simulink model "EngPrt_TrqLimPTO1"  (R2016b)
settings: configuration reference "CodeGenConfigSet" (kept outside this file)
values from neighbouring files (symbols this model uses):
  EngPrt_facPTOLim0_CUR = Calibration.Parameter    [init_EngPrt_TrqLimPTO.m]    (also in init_EngPrt_TrqLimPTO_SIL.m = Simulink.Parameter)
  EngPrt_facPTOLim0_CURX = Calibration.Parameter    [init_EngPrt_TrqLimPTO.m]    (also in init_EngPrt_TrqLimPTO_SIL.m = Simulink.Parameter)
  EngPrt_facPTOLim1_CUR = Calibration.Parameter    [init_EngPrt_TrqLimPTO.m]    (also in init_EngPrt_TrqLimPTO_SIL.m = Simulink.Parameter)
  EngPrt_facPTOLim1_CURX = Calibration.Parameter    [init_EngPrt_TrqLimPTO.m]    (also in init_EngPrt_TrqLimPTO_SIL.m = Simulink.Parameter)
  EngPrt_facPTOLim2_CUR = Calibration.Parameter    [init_EngPrt_TrqLimPTO.m]    (also in init_EngPrt_TrqLimPTO_SIL.m = Simulink.Parameter)
  EngPrt_facPTOLim2_CURX = Calibration.Parameter    [init_EngPrt_TrqLimPTO.m]    (also in init_EngPrt_TrqLimPTO_SIL.m = Simulink.Parameter)
  EngPrt_facPTOLim3_CUR = Calibration.Parameter    [init_EngPrt_TrqLimPTO.m]    (also in init_EngPrt_TrqLimPTO_SIL.m = Simulink.Parameter)
  EngPrt_facPTOLim3_CURX = Calibration.Parameter    [init_EngPrt_TrqLimPTO.m]    (also in init_EngPrt_TrqLimPTO_SIL.m = Simulink.Parameter)
  EngPrt_facPTOLim4_CUR = Calibration.Parameter    [init_EngPrt_TrqLimPTO.m]    (also in init_EngPrt_TrqLimPTO_SIL.m = Simulink.Parameter)
  EngPrt_facPTOLim4_CURX = Calibration.Parameter    [init_EngPrt_TrqLimPTO.m]    (also in init_EngPrt_TrqLimPTO_SIL.m = Simulink.Parameter)
settings Model: Creator=lenovo  LastModifiedBy=lenovo
settings ConfigSetRef: SourceLocation=Base Workspace

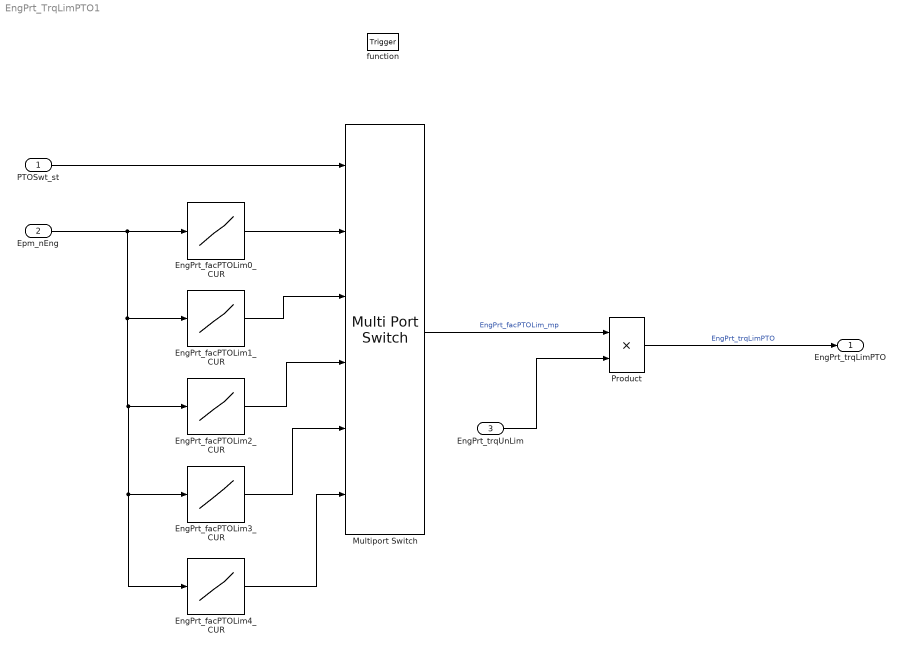
== system EngPrt_TrqLimPTO1 ==
  PTOSwt_st : Inport  Description=Power Take-off switch current state for a specific input voltage  OutMin=0  OutMax=255  OutDataTypeStr=State_uint8
  Epm_nEng : Inport  Tag=rpm  Description=Engine speed  Port=2  OutMin=0  OutMax=6000  OutDataTypeStr=EngSpeed_rpm
  EngPrt_trqUnLim : Inport  Tag=Nm  Description=Enabled torque from the maximum power manager  Port=3  OutMin=-3276.8  OutMax=3276.7  OutDataTypeStr=Trq_Nm
  function : TriggerPort  TriggerType=function-call  VariantControl=Variant
  EngPrt_facPTOLim0_CUR : Lookup_n-D  NumberOfTableDimensions=1  BreakpointsForDimension1=EngPrt_facPTOLim0_CURX  BreakpointsForDimension1DataTypeStr=Inherit: Inherit from 'Breakpoint data'  IndexSearchMethod=Linear search  Table=EngPrt_facPTOLim0_CUR  TableDataTypeStr=Inherit: Inherit from 'Table data'  ExtrapMethod=Clip  InternalRulePriority=Speed  OutDataTypeStr=Inherit: Inherit from 'Table data'  RndMeth=Simplest  SaturateOnIntegerOverflow=on
  EngPrt_facPTOLim1_CUR : Lookup_n-D  NumberOfTableDimensions=1  BreakpointsForDimension1=EngPrt_facPTOLim1_CURX  BreakpointsForDimension1DataTypeStr=Inherit: Inherit from 'Breakpoint data'  IndexSearchMethod=Linear search  Table=EngPrt_facPTOLim1_CUR  TableDataTypeStr=Inherit: Inherit from 'Table data'  ExtrapMethod=Clip  InternalRulePriority=Speed  OutDataTypeStr=Inherit: Inherit from 'Table data'  RndMeth=Simplest  SaturateOnIntegerOverflow=on
  EngPrt_facPTOLim2_CUR : Lookup_n-D  NumberOfTableDimensions=1  BreakpointsForDimension1=EngPrt_facPTOLim2_CURX  IndexSearchMethod=Linear search  Table=EngPrt_facPTOLim2_CUR  ExtrapMethod=Clip  InternalRulePriority=Speed  OutDataTypeStr=Inherit: Inherit from 'Table data'  RndMeth=Simplest  SaturateOnIntegerOverflow=on
  EngPrt_facPTOLim3_CUR : Lookup_n-D  NumberOfTableDimensions=1  BreakpointsForDimension1=EngPrt_facPTOLim3_CURX  BreakpointsForDimension1DataTypeStr=Inherit: Inherit from 'Breakpoint data'  IndexSearchMethod=Linear search  Table=EngPrt_facPTOLim3_CUR  TableDataTypeStr=Inherit: Inherit from 'Table data'  ExtrapMethod=Clip  InternalRulePriority=Speed  OutDataTypeStr=Inherit: Inherit from 'Table data'  RndMeth=Simplest  SaturateOnIntegerOverflow=on
  EngPrt_facPTOLim4_CUR : Lookup_n-D  NumberOfTableDimensions=1  BreakpointsForDimension1=EngPrt_facPTOLim4_CURX  BreakpointsForDimension1DataTypeStr=Inherit: Inherit from 'Breakpoint data'  IndexSearchMethod=Linear search  Table=EngPrt_facPTOLim4_CUR  TableDataTypeStr=Inherit: Inherit from 'Table data'  ExtrapMethod=Clip  InternalRulePriority=Speed  OutDataTypeStr=Inherit: Inherit from 'Table data'  RndMeth=Simplest  SaturateOnIntegerOverflow=on
  Multiport Switch : MultiPortSwitch  DataPortOrder=Zero-based contiguous  Inputs=5  OutDataTypeStr=Inherit: Inherit via back propagation
  Product : Product  OutDataTypeStr=Inherit: Inherit via back propagation
  EngPrt_trqLimPTO : Outport  Tag=Nm  Description=Torque limitation value from PTO state  OutMin=-3276.8  OutMax=3276.7  OutDataTypeStr=Trq_Nm
  wires:
  Product/1 -> EngPrt_trqLimPTO/1  "EngPrt_trqLimPTO"
  PTOSwt_st/1 -> Multiport Switch/1
  Epm_nEng/1 -> EngPrt_facPTOLim4_CUR/1, EngPrt_facPTOLim3_CUR/1, EngPrt_facPTOLim2_CUR/1, EngPrt_facPTOLim1_CUR/1, EngPrt_facPTOLim0_CUR/1
  EngPrt_facPTOLim0_CUR/1 -> Multiport Switch/2
  EngPrt_facPTOLim1_CUR/1 -> Multiport Switch/3
  EngPrt_facPTOLim2_CUR/1 -> Multiport Switch/4
  EngPrt_facPTOLim3_CUR/1 -> Multiport Switch/5
  EngPrt_facPTOLim4_CUR/1 -> Multiport Switch/6
  Multiport Switch/1 -> Product/1  "EngPrt_facPTOLim_mp"
  EngPrt_trqUnLim/1 -> Product/2
